simulink model "multi_gadget"  (Simulink 6.6)
settings: Solver=ode3  SolverMode=SingleTasking  StartTime=0.0  StopTime=Inf  FixedStep=.001  RelTol=1e-3
libraries: xpclib x7, xpcnilib x5, limblab x2, simulink x2
settings Model: Creator=Selket  LastModifiedBy=limblab  BufferReuse=off
settings OptimizationCC: BlockReduction=off  OptimizeBlockIOStorage=off  BufferReuse=off  ExpressionFolding=off  LocalBlockOutputs=off
settings RTWCC: SystemTargetFile=xpctarget.tlc  TemplateMakefile=xpc_default_tmf  Description=xPC Target  ProcessScript=xpctarget_make_rtw_hook
settings xpcTargetCC: TargetFcnLib=ansi_tfl_tmw.mat  GenFloatMathFcnCalls=ANSI_C  PortableWordSizes=off

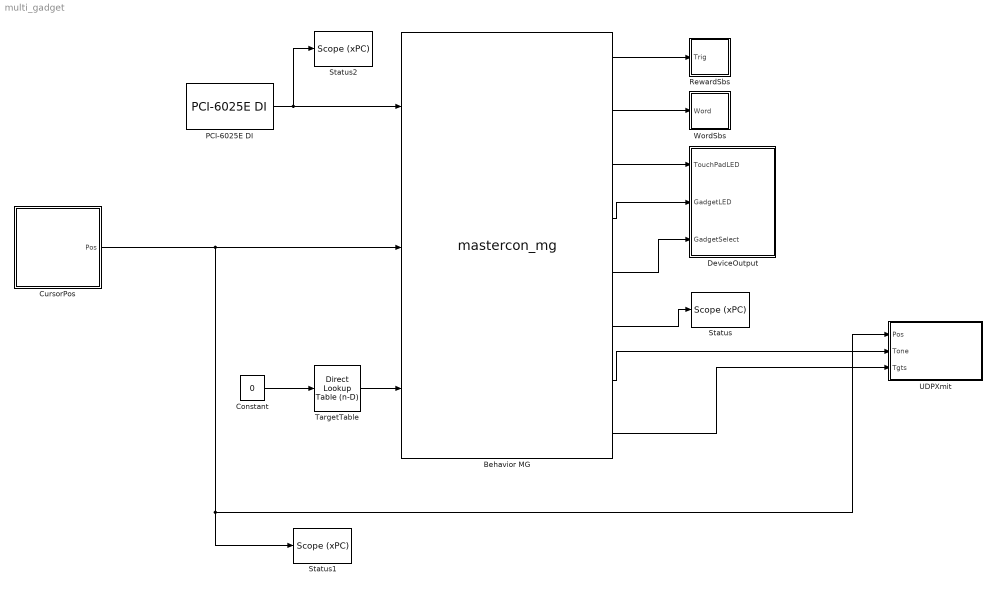
== system multi_gadget ==
  Behavior MG : S-Function  FunctionName=mastercon_mg  Parameters=3 .25 .75 1 3 10 1 1 1 0 0 0 0
      mask Display:
      | disp('Master Control\nMulti-Gadget')
      | port_label('input',1,'touch pad')
      | port_label('input',2,'cursor')
      | port_label('input',3,'target list')
      | port_label('output',1,'Reward')
      | port_label('output',2,'Word')
      | port_label('output',3,'TP LED')
      | port_label('output',4,'Gadget LED')
      | port_label('output',5,'Gadget Select')
      | port_label('output',6,'Status')
      | port_label('output',7,'Tone')
      | port_label('output',8,'Targets')
  Constant : Constant  Value=0
  CursorPos : Subsystem
  DeviceOutput : Subsystem
  PCI-6025E DI : xpcnilib/Digital Input/PCI-6025E DI  channel=[3]  sampletime=0.001  slot=-1
  RewardSbs : Subsystem
  Status : xpclib/Misc./Scope (xPC)   SystemSampleTime=-1  scopeno=1  scopetype=Target  autostart=on  viewmode=Numerical  formatstr='%6.0f tgt_index,%6.0f num_tgt,%6.0f num gdt in use,%6.0f tgt_id'  grid=on  ylimits=[-10,10]  nosamples=10  noprepostsamples=0  interleave=10  triggermode=FreeRun  triggersignal=1  triggerlevel=0.0  triggerslope=Either  triggerscope=1  triggersample=0  filename=data.dat  mode=Lazy  writesize=512  autorestart=off
  Status1 : xpclib/Misc./Scope (xPC)   SystemSampleTime=-1  scopeno=2  scopetype=Target  autostart=on  viewmode=Numerical  formatstr=' %6.6f X, %6.6f Y'  grid=on  ylimits=[-10,10]  nosamples=10  noprepostsamples=0  interleave=10  triggermode=FreeRun  triggersignal=1  triggerlevel=0.0  triggerslope=Either  triggerscope=1  triggersample=0  filename=data.dat  mode=Lazy  writesize=512  autorestart=off
  Status2 : xpclib/Misc./Scope (xPC)   SystemSampleTime=-1  scopeno=3  scopetype=Target  autostart=on  viewmode=Numerical  formatstr='%6.0f Touch Pad'  grid=on  ylimits=[-10,10]  nosamples=10  noprepostsamples=0  interleave=10  triggermode=FreeRun  triggersignal=1  triggerlevel=0.0  triggerslope=Either  triggerscope=1  triggersample=0  filename=data.dat  mode=Lazy  writesize=512  autorestart=off
  TargetTable : simulink/Lookup Tables/Direct Lookup Table (n-D)  maskTabDims=2  explicitNumDims=1  outDims=Column  tabIsInput=off  mxTable=[0.75 1.25 2; 0.5 0.5 0.75; 0 0 0; 2 3 4]  clipFlag=Warning  samptime=-1
  UDPXmit : Subsystem
  WordSbs : Subsystem
  wires:
  Behavior MG/2 -> WordSbs/1(Word)
  Behavior MG/3 -> DeviceOutput/1(TouchPadLED)
  Behavior MG/4 -> DeviceOutput/2(GadgetLED)
  Behavior MG/5 -> DeviceOutput/3(GadgetSelect)
  Behavior MG/6 -> Status/1
  Behavior MG/1 -> RewardSbs/1(Trig)
  Behavior MG/8 -> UDPXmit/3(Tgts)
  Behavior MG/7 -> UDPXmit/2(Tone)
  PCI-6025E DI/1 -> Behavior MG/1, Status2/1
  TargetTable/1 -> Behavior MG/3
  CursorPos/1(Pos) -> Behavior MG/2, UDPXmit/1(Pos), Status1/1
  Constant/1 -> TargetTable/1

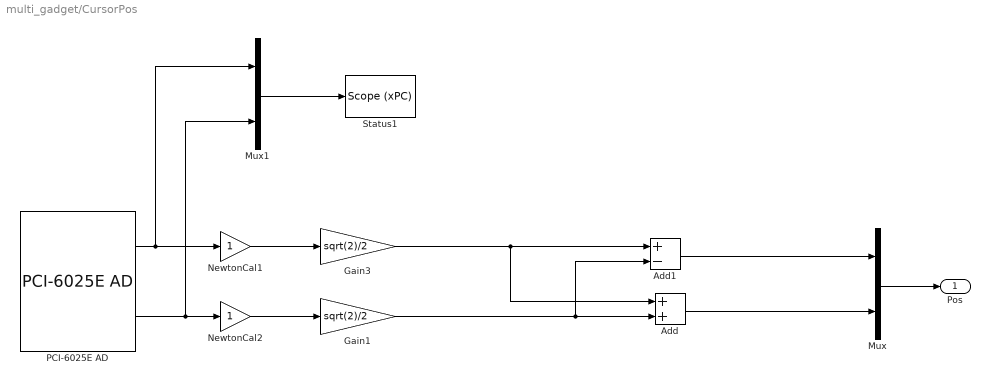
== system multi_gadget/CursorPos ==
  Add : Sum  OutScaling=2^-10
  Add1 : Sum  Inputs=+-  OutScaling=2^-10
  Gain1 : Gain  Gain=sqrt(2)/2
  Gain3 : Gain  Gain=sqrt(2)/2
  Mux : Mux  Inputs=2
  Mux1 : Mux  Inputs=2
  NewtonCal1 : Gain
  NewtonCal2 : Gain
  PCI-6025E AD : xpcnilib/A//D/PCI-6025E AD  channel=[9 10]  range=[-10]  coupling=[0]  sampletime=0.001  slot=-1
  Status1 : xpclib/Misc./Scope (xPC)   SystemSampleTime=-1  scopeno=4  scopetype=Target  autostart=on  viewmode=Numerical  formatstr=' %6.6f Raw 1, %6.6f Raw 2'  grid=on  ylimits=[-10,10]  nosamples=10  noprepostsamples=0  interleave=10  triggermode=FreeRun  triggersignal=1  triggerlevel=0.0  triggerslope=Either  triggerscope=1  triggersample=0  filename=data.dat  mode=Lazy  writesize=512  autorestart=off
  Pos : Outport
  wires:
  PCI-6025E AD/1 -> NewtonCal1/1, Mux1/1
  PCI-6025E AD/2 -> NewtonCal2/1, Mux1/2
  Mux/1 -> Pos/1
  NewtonCal1/1 -> Gain3/1
  NewtonCal2/1 -> Gain1/1
  Gain3/1 -> Add/1, Add1/1
  Gain1/1 -> Add/2, Add1/2
  Add/1 -> Mux/2
  Add1/1 -> Mux/1
  Mux1/1 -> Status1/1

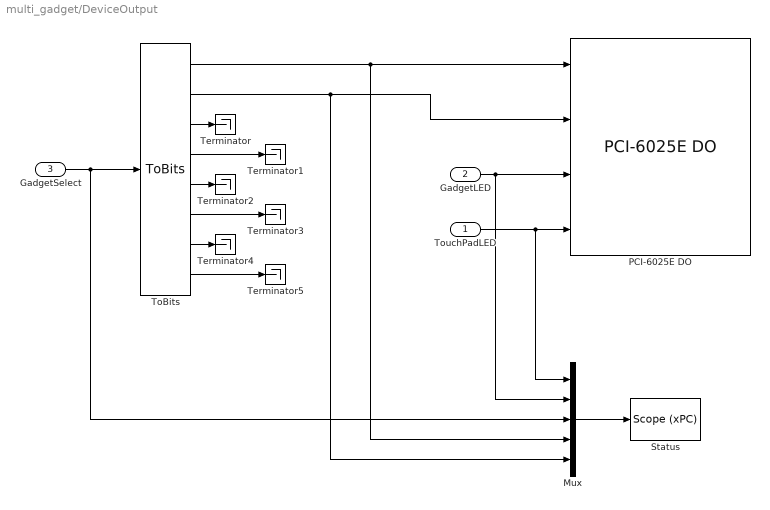
== system multi_gadget/DeviceOutput ==
  TouchPadLED : Inport
  GadgetLED : Inport  Port=2
  GadgetSelect : Inport  Port=3
  Mux : Mux  Inputs=5
  PCI-6025E DO : xpcnilib/Digital Output/PCI-6025E DO  channel=[4 5 6 8]  reset=[1]  initValue=[0]  sampletime=0.001  slot=-1
  Status : xpclib/Misc./Scope (xPC)   SystemSampleTime=-1  scopeno=5  scopetype=Target  autostart=on  viewmode=Numerical  formatstr='%6.0f TP_LED,%6.0f Gdt_LED,%6.0f Gdt_Select,%6.0f Gdt_bit0,%6.0f Gdt_bit1'  grid=on  ylimits=[-10,10]  nosamples=10  noprepostsamples=0  interleave=10  triggermode=FreeRun  triggersignal=1  triggerlevel=0.0  triggerslope=Either  triggerscope=1  triggersample=0  filename=data.dat  mode=Lazy  writesize=512  autorestart=off
  Terminator{,1..5} (6 alike) : Terminator
  ToBits : limblab/ToBits
  wires:
  GadgetLED/1 -> PCI-6025E DO/3, Mux/2
  TouchPadLED/1 -> PCI-6025E DO/4, Mux/1
  GadgetSelect/1 -> ToBits/1, Mux/3
  ToBits/1 -> PCI-6025E DO/1, Mux/4
  ToBits/2 -> PCI-6025E DO/2, Mux/5
  ToBits/4 -> Terminator1/1
  ToBits/3 -> Terminator/1
  ToBits/5 -> Terminator2/1
  ToBits/6 -> Terminator3/1
  ToBits/7 -> Terminator4/1
  ToBits/8 -> Terminator5/1
  Mux/1 -> Status/1

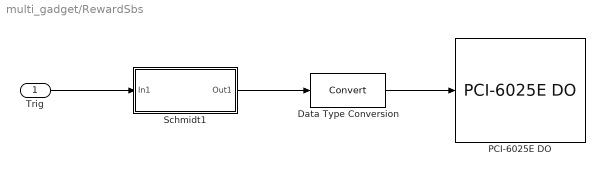
== system multi_gadget/RewardSbs ==
  Trig : Inport
  Data Type Conversion : DataTypeConversion
  PCI-6025E DO : xpcnilib/Digital Output/PCI-6025E DO  channel=[2]  reset=[1]  initValue=[0]  sampletime=0.001  slot=-1
  Schmidt1 : Subsystem  mask(Schmidt Trigger){Time=.3}
      mask help: Creates an output pulse of the specified time in seconds when trig goes high
      mask Help: Creates an output pulse of the specified time in seconds when trig goes high
      mask Display:
      | port_label('output',1,'out')
      | port_label('input',1,'trig')
      | fprintf('t = %.2f',Time)
  wires:
  Trig/1 -> Schmidt1/1(In1)
  Data Type Conversion/1 -> PCI-6025E DO/1
  Schmidt1/1(Out1) -> Data Type Conversion/1

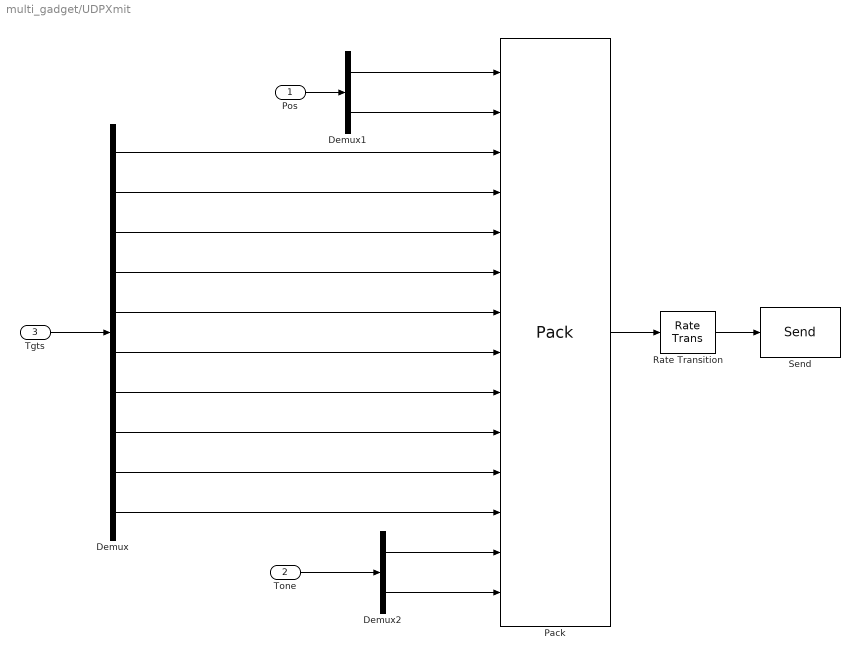
== system multi_gadget/UDPXmit ==
  Pos : Inport
  Tone : Inport  Port=2
  Tgts : Inport  Port=3
  Demux : Demux  Outputs=10
  Demux1 : Demux  Outputs=2
  Demux2 : Demux  Outputs=2
  Pack : xpclib/UDP/Pack  datatypes={'double', 'double','double','double','double','double','double','double','double','double','double','double','double','double'}  byteAlign=1
  Rate Transition : RateTransition
  Send : xpclib/UDP/Send  ipAddress=192.168.0.2  ipPort=25000  localPort=-1  sampletime=.02
  wires:
  Rate Transition/1 -> Send/1
  Pack/1 -> Rate Transition/1
  Demux/10 -> Pack/12
  Demux/9 -> Pack/11
  Demux/8 -> Pack/10
  Demux/7 -> Pack/9
  Demux/6 -> Pack/8
  Demux/5 -> Pack/7
  Demux/4 -> Pack/6
  Demux/3 -> Pack/5
  Demux/2 -> Pack/4
  Demux/1 -> Pack/3
  Demux1/1 -> Pack/1
  Demux1/2 -> Pack/2
  Pos/1 -> Demux1/1
  Demux2/1 -> Pack/13
  Demux2/2 -> Pack/14
  Tone/1 -> Demux2/1
  Tgts/1 -> Demux/1

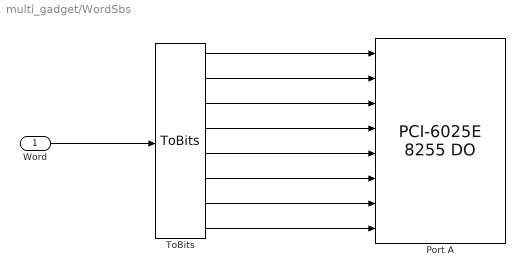
== system multi_gadget/WordSbs ==
  Word : Inport
  Port A : xpcnilib/Digital Output/PCI-6025E 8255 DO  channel=1:8  port=A  reset=[1]  initValue=[0]  chip=1  sampletime=-1  slot=[0 16]
  ToBits : limblab/ToBits
  wires:
  Word/1 -> ToBits/1
  ToBits/1 -> Port A/1
  ToBits/2 -> Port A/2
  ToBits/3 -> Port A/3
  ToBits/4 -> Port A/4
  ToBits/5 -> Port A/5
  ToBits/6 -> Port A/6
  ToBits/7 -> Port A/7
  ToBits/8 -> Port A/8

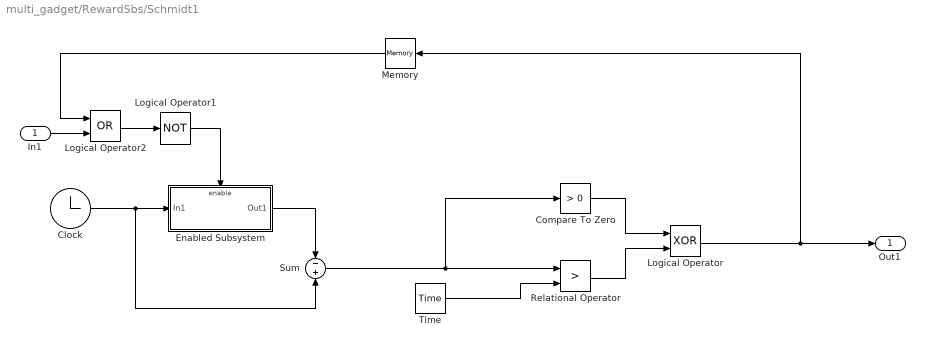
== system multi_gadget/RewardSbs/Schmidt1 ==
  In1 : Inport
  Clock : Clock
  Compare To Zero : simulink/Logic and Bit Operations/Compare To Zero  SystemSampleTime=-1  relop=>  LogicOutDataTypeMode=uint8  ZeroCross=off
  Enabled Subsystem : Subsystem  TreatAsAtomicUnit=on
  Logical Operator : Logic  Operator=XOR  AllPortsSameDT=off  OutDataTypeMode=Boolean  SampleTime=.001
  Logical Operator1 : Logic  Operator=NOT  AllPortsSameDT=off  OutDataTypeMode=Boolean
  Logical Operator2 : Logic  Operator=OR  AllPortsSameDT=off  OutDataTypeMode=Boolean  SampleTime=.001
  Memory : Memory  Orientation=left
  Relational Operator : RelationalOperator  Operator=>  LogicOutDataTypeMode=Boolean
  Sum : Sum  Inputs=-+
  Time : Constant  Value=Time
  Out1 : Outport
  wires:
  Clock/1 -> Enabled Subsystem/1(In1), Sum/2
  Enabled Subsystem/1(Out1) -> Sum/1
  Sum/1 -> Compare To Zero/1, Relational Operator/1
  Time/1 -> Relational Operator/2
  Compare To Zero/1 -> Logical Operator/1
  Relational Operator/1 -> Logical Operator/2
  Logical Operator1/1 -> Enabled Subsystem/Enable
  Logical Operator/1 -> Out1/1, Memory/1
  In1/1 -> Logical Operator2/2
  Logical Operator2/1 -> Logical Operator1/1
  Memory/1 -> Logical Operator2/1

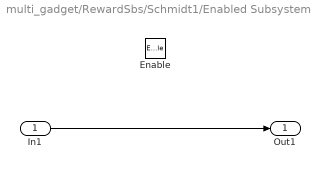
== system multi_gadget/RewardSbs/Schmidt1/Enabled Subsystem ==
  In1 : Inport
  Enable : EnablePort
  Out1 : Outport
  wires:
  In1/1 -> Out1/1
